simulink model "VODARNA_SPACE_TURBO_GENERATOR"  (R2012b)
settings: Solver=ode45  StartTime=0.0  StopTime=100  MaxStep=1e-2  MinStep=1e-3  RelTol=1e-3
values from neighbouring files (symbols this model uses):
  C1 = 25    [iniFINAL.m]
  C2 = 25    [iniFINAL.m]
  C3 = 500    [iniFINAL.m]
  CT = .2    (= 0.2)    [iniFINAL.m]
  g = 2    [iniFINAL.m]
  G = 13.5    [iniFINAL.m]
  G2 = 0.4    [iniFINAL.m]
  I = 5    [iniFINAL.m]
  R1 = 6    [iniFINAL.m]
  R2 = 2    [iniFINAL.m]
  R5 = 1.5    [iniFINAL.m]
  RV1 = 2    [iniFINAL.m]
  RV2 = 2    [iniFINAL.m]
settings Model: Creator=SerzaNT  LastModifiedBy=SerzaNT

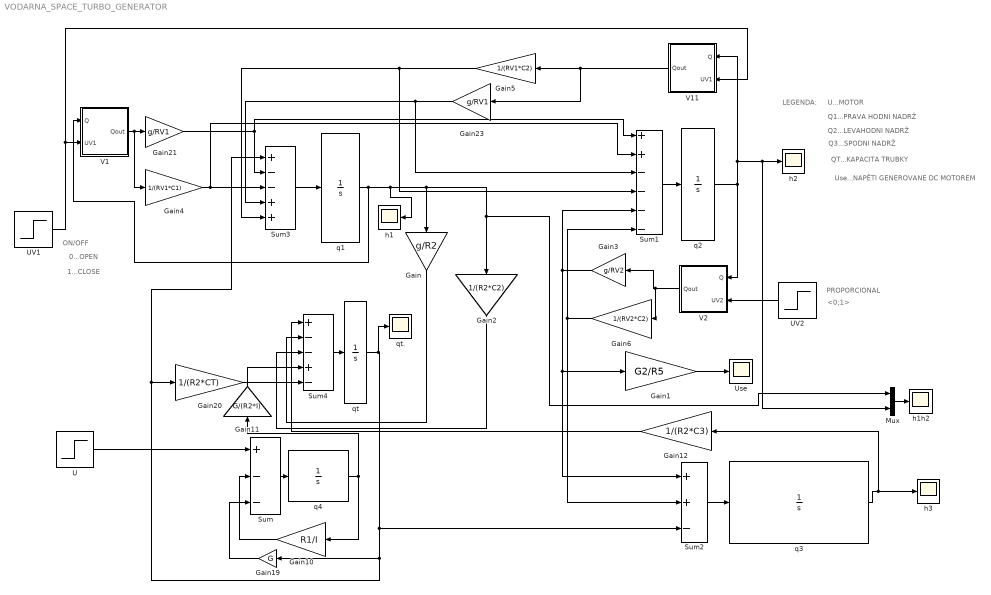
== system VODARNA_SPACE_TURBO_GENERATOR ==
  note: <0;1>
  note: PROPORCIONAL
  note: 1...CLOSE
  note: 0...OPEN
  note: ON/OFF
  note: Use...NAPĚTI GENEROVANE DC MOTOREM
  note: QT...KAPACITA TRUBKY
  note: LEGENDA:
  note: U...MOTOR
  note: Q1...PRAVA HODNI NADRŽ
  note: Q2...LEVAHODNI NADRŽ
  note: Q3...SPODNI NADRŽ
  Gain : Gain  Gain=g/R2
  Gain1 : Gain  Gain=G2/R5
  Gain10 : Gain  Gain=R1/I
  Gain11 : Gain  Gain=G/(R2*I)
  Gain12 : Gain  Gain=1/(R2*C3)
  Gain19 : Gain  Gain=G
  Gain2 : Gain  Gain=1/(R2*C2)
  Gain20 : Gain  Gain=1/(R2*CT)
  Gain21 : Gain  Gain=g/RV1
  Gain23 : Gain  Gain=g/RV1
  Gain3 : Gain  Gain=g/RV2
  Gain4 : Gain  Gain=1/(RV1*C1)
  Gain5 : Gain  Gain=1/(RV1*C2)
  Gain6 : Gain  Gain=1/(RV2*C2)
  Mux : Mux  Inputs=2
  Sum : Sum  Inputs=+--
  Sum1 : Sum  Inputs=++----
  Sum2 : Sum  Inputs=++-
  Sum3 : Sum  Inputs=+--++
  Sum4 : Sum  Inputs=+--+-
  U : Step  Time=30  Before=66  After=0  SampleTime=0
  UV1 : Step  Time=30  Before=1  After=0  SampleTime=0
  UV2 : Step  Time=60  Before=1  After=0  SampleTime=0
  Use : Scope
      settings: SaveName=h
  V1 : Subsystem
      mask Display: image(imread('V1.png'))
  V11 : Subsystem
      mask Display: image(imread('V1.png'))
  V2 : Subsystem
      mask Display: image(imread('V2.png'))
  h1 : Scope
  h1h2 : Scope
      settings: TimeRange=60  YMin=72.7935  YMax=72.794
  h2 : Scope
      settings: SaveName=ScopeData2
  h3 : Scope
      settings: SaveName=h1
  q1 : Integrator  UpperSaturationLimit=C1  LowerSaturationLimit=0
      mask Display: image(imread('Q1.png'))
  q2 : Integrator  UpperSaturationLimit=C2  LowerSaturationLimit=0
      mask Display: image(imread('Q2.png'))
  q3 : Integrator  InitialCondition=50  UpperSaturationLimit=C3  LowerSaturationLimit=0
      mask Display: image(imread('Q3.png'))
  q4 : Integrator
      mask Display: image(imread('P.png'))
  qt : Integrator  UpperSaturationLimit=CT  LowerSaturationLimit=0
      mask Display: image(imread('T.png'))
  qt. : Scope
      settings: SaveName=ScopeData3
  wires:
  Sum1/1 -> q2/1
  Sum2/1 -> q3/1
  q3/1 -> Gain12/1, h3/1
  Mux/1 -> h1h2/1
  Sum/1 -> q4/1
  Sum3/1 -> q1/1
  U/1 -> Sum/1
  q4/1 -> Gain11/1, Gain10/1
  Gain10/1 -> Sum/2
  Sum4/1 -> qt/1
  qt/1 -> Sum2/3, Gain20/1, Sum3/1, Gain19/1, qt./1
  Gain19/1 -> Sum/3
  Gain12/1 -> Sum4/1
  q1/1 -> h1/1, Gain/1, Mux/1, Gain2/1, V1/1(Q)
  Gain/1 -> Sum4/2
  Gain2/1 -> Sum4/3
  Gain11/1 -> Sum4/4
  Gain20/1 -> Sum4/5
  Gain21/1 -> Sum3/2, Sum1/1
  Gain4/1 -> Sum1/2, Sum3/3
  q2/1 -> V2/1(Q), V11/1(Q), Mux/2, h2/1
  Gain23/1 -> Sum1/3, Sum3/4
  V11/1(Qout) -> Gain23/1, Gain5/1
  Gain3/1 -> Sum1/5, Gain1/1, Sum2/1
  Gain6/1 -> Sum2/2, Sum1/6
  Gain1/1 -> Use/1
  V1/1(Qout) -> Gain4/1, Gain21/1
  Gain5/1 -> Sum1/4, Sum3/5
  UV1/1 -> V11/2(UV1), V1/2(UV1)
  V2/1(Qout) -> Gain6/1, Gain3/1
  UV2/1 -> V2/2(UV2)

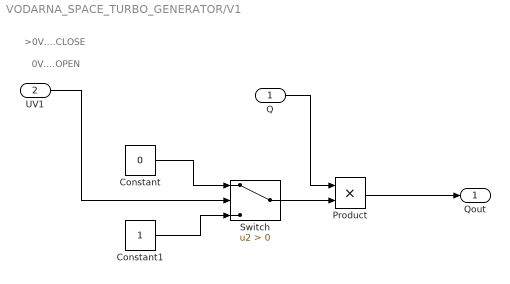
== system VODARNA_SPACE_TURBO_GENERATOR/V1 ==
  note: >0V....CLOSE
  note: 0V....OPEN
  Q : Inport
  Constant : Constant  Value=0
  Constant1 : Constant
  Product : Product  RndMeth=Zero
  Switch : Switch  Criteria=u2 > Threshold
  UV1 : Inport  Port=2
  Qout : Outport
  wires:
  Q/1 -> Product/1
  Product/1 -> Qout/1
  UV1/1 -> Switch/2
  Constant/1 -> Switch/1
  Constant1/1 -> Switch/3
  Switch/1 -> Product/2

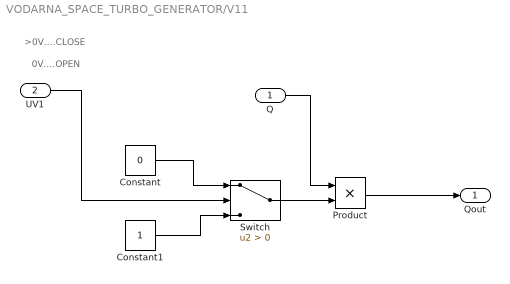
== system VODARNA_SPACE_TURBO_GENERATOR/V11 ==
  note: 0V....OPEN
  note: >0V....CLOSE
  Q : Inport
  UV1 : Inport  Port=2
  Constant : Constant  Value=0
  Constant1 : Constant
  Product : Product  RndMeth=Zero
  Switch : Switch  Criteria=u2 > Threshold
  Qout : Outport
  wires:
  Switch/1 -> Product/2
  Constant1/1 -> Switch/3
  Constant/1 -> Switch/1
  UV1/1 -> Switch/2
  Product/1 -> Qout/1
  Q/1 -> Product/1

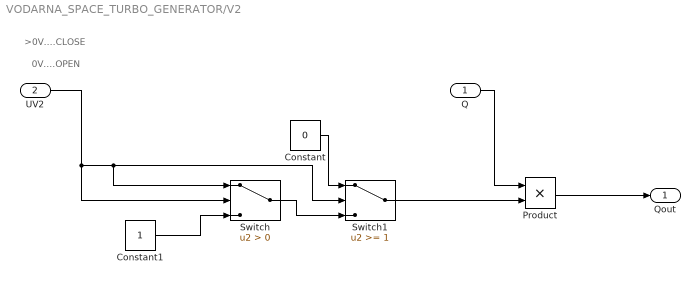
== system VODARNA_SPACE_TURBO_GENERATOR/V2 ==
  note: >0V....CLOSE
  note: 0V....OPEN
  Q : Inport
  UV2 : Inport  Port=2
  Constant : Constant  Value=0
  Constant1 : Constant
  Product : Product  RndMeth=Zero
  Switch : Switch  Criteria=u2 > Threshold
  Switch1 : Switch  Threshold=1
  Qout : Outport
  wires:
  Q/1 -> Product/1
  Product/1 -> Qout/1
  UV2/1 -> Switch/2, Switch/1, Switch1/2
  Constant1/1 -> Switch/3
  Constant/1 -> Switch1/1
  Switch/1 -> Switch1/3
  Switch1/1 -> Product/2
